simulink model "jplsetispec_thresh_rev003"  (Simulink 6.2)
settings: Solver=ode45  StartTime=0.0  StopTime=100  RelTol=1e-3
libraries: xbsIndex_r3 x776, xps_library x53, casper_library x4
(part 4 of 5)

== system jplsetispec_thresh_rev003/in/ct_pole2_snapshot/negedge ==
  In : Inport  Port=1  LatchInput=off
  Delay : xbsIndex_r3/Delay  latency=1  reg_retiming=off  explicit_period=off  period=1  en=off  accept_only_valid=off  init_zero=on  dbl_ovrd=off  show_param=off
      settings: xl_area=[0, 0, 0, 0, 0, 0, 0]
  Inverter : xbsIndex_r3/Inverter  latency=0  explicit_period=off  period=1  en=off  dbl_ovrd=off  show_param=off
      settings: xl_area=[0, 0, 0, 0, 0, 0, 0]
  Logical : xbsIndex_r3/Logical  logical_function=AND  inputs=2  precision=Full  arith_type=Unsigned  n_bits=8  bin_pt=2  align_bp=on  latency=0  explicit_period=off  period=1  en=off  dbl_ovrd=off  show_param=off
      settings: xl_area=[0, 0, 0, 0, 0, 0, 0]
  Out : Outport
  wires:
  Logical/1 -> Out/1
  In/1 -> Delay/1, Inverter/1
  Delay/1 -> Logical/1
  Inverter/1 -> Logical/2

== system jplsetispec_thresh_rev003/in/ct_pole2_snapshot/posedge ==
  In : Inport  Port=1  LatchInput=off
  Delay : xbsIndex_r3/Delay  latency=1  reg_retiming=off  explicit_period=off  period=1  en=off  accept_only_valid=off  init_zero=on  dbl_ovrd=off  show_param=off
      settings: xl_area=[0, 0, 0, 0, 0, 0, 0]
  Inverter : xbsIndex_r3/Inverter  latency=0  explicit_period=off  period=1  en=off  dbl_ovrd=off  show_param=off
      settings: xl_area=[0, 0, 0, 0, 0, 0, 0]
  Logical : xbsIndex_r3/Logical  logical_function=AND  inputs=2  precision=Full  arith_type=Unsigned  n_bits=8  bin_pt=2  align_bp=on  latency=0  explicit_period=off  period=1  en=off  dbl_ovrd=off  show_param=off
      settings: xl_area=[0, 0, 0, 0, 0, 0, 0]
  Out : Outport
  wires:
  Delay/1 -> Inverter/1
  Inverter/1 -> Logical/1
  In/1 -> Delay/1, Logical/2
  Logical/1 -> Out/1

== system jplsetispec_thresh_rev003/in/ct_pole2_snapshot/posedge1 ==
  In : Inport  Port=1  LatchInput=off
  Delay : xbsIndex_r3/Delay  latency=1  reg_retiming=off  explicit_period=off  period=1  en=off  accept_only_valid=off  init_zero=on  dbl_ovrd=off  show_param=off
      settings: xl_area=[0, 0, 0, 0, 0, 0, 0]
  Inverter : xbsIndex_r3/Inverter  latency=0  explicit_period=off  period=1  en=off  dbl_ovrd=off  show_param=off
      settings: xl_area=[0, 0, 0, 0, 0, 0, 0]
  Logical : xbsIndex_r3/Logical  logical_function=AND  inputs=2  precision=Full  arith_type=Unsigned  n_bits=8  bin_pt=2  align_bp=on  latency=0  explicit_period=off  period=1  en=off  dbl_ovrd=off  show_param=off
      settings: xl_area=[0, 0, 0, 0, 0, 0, 0]
  Out : Outport
  wires:
  Logical/1 -> Out/1
  In/1 -> Logical/2, Delay/1
  Inverter/1 -> Logical/1
  Delay/1 -> Inverter/1

== system jplsetispec_thresh_rev003/in/fft_pole1_snapshot/freeze_cntr ==
  en : Inport  Port=1  LatchInput=off
  rst : Inport  Port=2  LatchInput=off
  Constant5 : xbsIndex_r3/Constant  const=2^CounterBits - 1  equ=P=C  arith_type=Unsigned  n_bits=CounterBits  bin_pt=0  opselect=C  inp2=PCIN>>17  opr=+  inp1=P  carry=CIN  iostate=0  explicit_period=off  period=1  dbl_ovrd=off
  Counter3 : xbsIndex_r3/Counter  cnt_type=Free Running  n_bits=CounterBits  bin_pt=0  arith_type=Unsigned  start_count=0  cnt_to=1023  cnt_by_val=1  operation=Up  explicit_period=on  period=1  load_pin=off  rst=on  en=on  dbl_ovrd=off  show_param=off  use_rpm=on  gen_core=off
      settings: xl_area=[0, 0, 0, 0, 0, 0, 0]
  Inverter : xbsIndex_r3/Inverter  latency=0  explicit_period=off  period=1  en=off  dbl_ovrd=off  show_param=off
      settings: xl_area=[0, 0, 0, 0, 0, 0, 0]
  Logical1 : xbsIndex_r3/Logical  logical_function=AND  inputs=2  precision=Full  arith_type=Unsigned  n_bits=8  bin_pt=2  align_bp=on  latency=0  explicit_period=off  period=1  en=off  dbl_ovrd=off  show_param=off
      settings: xl_area=[0, 0, 0, 0, 0, 0, 0]
  Logical5 : xbsIndex_r3/Logical  logical_function=AND  inputs=2  precision=Full  arith_type=Unsigned  n_bits=8  bin_pt=2  align_bp=on  latency=0  explicit_period=off  period=1  en=off  dbl_ovrd=off  show_param=off
      settings: xl_area=[0, 0, 0, 0, 0, 0, 0]
  Relational5 : xbsIndex_r3/Relational  mode=a!=b  latency=0  explicit_period=off  period=1  en=off  dbl_ovrd=off  show_param=off
      settings: xl_area=[0, 0, 0, 0, 0, 0, 0]
  addr : Outport
  we : Outport  Port=2
  wires:
  Logical1/1 -> we/1
  Inverter/1 -> Logical1/1
  Counter3/1 -> addr/1, Relational5/1
  Constant5/1 -> Relational5/2
  Relational5/1 -> Logical5/2
  en/1 -> Logical5/1
  Logical5/1 -> Logical1/2, Counter3/2
  rst/1 -> Inverter/1, Counter3/1

== system jplsetispec_thresh_rev003/in/fft_pole1_snapshot/negedge ==
  In : Inport  Port=1  LatchInput=off
  Delay : xbsIndex_r3/Delay  latency=1  reg_retiming=off  explicit_period=off  period=1  en=off  accept_only_valid=off  init_zero=on  dbl_ovrd=off  show_param=off
      settings: xl_area=[0, 0, 0, 0, 0, 0, 0]
  Inverter : xbsIndex_r3/Inverter  latency=0  explicit_period=off  period=1  en=off  dbl_ovrd=off  show_param=off
      settings: xl_area=[0, 0, 0, 0, 0, 0, 0]
  Logical : xbsIndex_r3/Logical  logical_function=AND  inputs=2  precision=Full  arith_type=Unsigned  n_bits=8  bin_pt=2  align_bp=on  latency=0  explicit_period=off  period=1  en=off  dbl_ovrd=off  show_param=off
      settings: xl_area=[0, 0, 0, 0, 0, 0, 0]
  Out : Outport
  wires:
  Inverter/1 -> Logical/2
  Delay/1 -> Logical/1
  In/1 -> Inverter/1, Delay/1
  Logical/1 -> Out/1

== system jplsetispec_thresh_rev003/in/fft_pole1_snapshot/posedge ==
  In : Inport  Port=1  LatchInput=off
  Delay : xbsIndex_r3/Delay  latency=1  reg_retiming=off  explicit_period=off  period=1  en=off  accept_only_valid=off  init_zero=on  dbl_ovrd=off  show_param=off
      settings: xl_area=[0, 0, 0, 0, 0, 0, 0]
  Inverter : xbsIndex_r3/Inverter  latency=0  explicit_period=off  period=1  en=off  dbl_ovrd=off  show_param=off
      settings: xl_area=[0, 0, 0, 0, 0, 0, 0]
  Logical : xbsIndex_r3/Logical  logical_function=AND  inputs=2  precision=Full  arith_type=Unsigned  n_bits=8  bin_pt=2  align_bp=on  latency=0  explicit_period=off  period=1  en=off  dbl_ovrd=off  show_param=off
      settings: xl_area=[0, 0, 0, 0, 0, 0, 0]
  Out : Outport
  wires:
  Logical/1 -> Out/1
  In/1 -> Logical/2, Delay/1
  Inverter/1 -> Logical/1
  Delay/1 -> Inverter/1

== system jplsetispec_thresh_rev003/in/fft_pole1_snapshot/posedge1 ==
  In : Inport  Port=1  LatchInput=off
  Delay : xbsIndex_r3/Delay  latency=1  reg_retiming=off  explicit_period=off  period=1  en=off  accept_only_valid=off  init_zero=on  dbl_ovrd=off  show_param=off
      settings: xl_area=[0, 0, 0, 0, 0, 0, 0]
  Inverter : xbsIndex_r3/Inverter  latency=0  explicit_period=off  period=1  en=off  dbl_ovrd=off  show_param=off
      settings: xl_area=[0, 0, 0, 0, 0, 0, 0]
  Logical : xbsIndex_r3/Logical  logical_function=AND  inputs=2  precision=Full  arith_type=Unsigned  n_bits=8  bin_pt=2  align_bp=on  latency=0  explicit_period=off  period=1  en=off  dbl_ovrd=off  show_param=off
      settings: xl_area=[0, 0, 0, 0, 0, 0, 0]
  Out : Outport
  wires:
  Delay/1 -> Inverter/1
  Inverter/1 -> Logical/1
  In/1 -> Delay/1, Logical/2
  Logical/1 -> Out/1

== system jplsetispec_thresh_rev003/in/fft_pole2_snapshot/freeze_cntr ==
  en : Inport  Port=1  LatchInput=off
  rst : Inport  Port=2  LatchInput=off
  Constant5 : xbsIndex_r3/Constant  const=2^CounterBits - 1  equ=P=C  arith_type=Unsigned  n_bits=CounterBits  bin_pt=0  opselect=C  inp2=PCIN>>17  opr=+  inp1=P  carry=CIN  iostate=0  explicit_period=off  period=1  dbl_ovrd=off
  Counter3 : xbsIndex_r3/Counter  cnt_type=Free Running  n_bits=CounterBits  bin_pt=0  arith_type=Unsigned  start_count=0  cnt_to=1023  cnt_by_val=1  operation=Up  explicit_period=on  period=1  load_pin=off  rst=on  en=on  dbl_ovrd=off  show_param=off  use_rpm=on  gen_core=off
      settings: xl_area=[0, 0, 0, 0, 0, 0, 0]
  Inverter : xbsIndex_r3/Inverter  latency=0  explicit_period=off  period=1  en=off  dbl_ovrd=off  show_param=off
      settings: xl_area=[0, 0, 0, 0, 0, 0, 0]
  Logical1 : xbsIndex_r3/Logical  logical_function=AND  inputs=2  precision=Full  arith_type=Unsigned  n_bits=8  bin_pt=2  align_bp=on  latency=0  explicit_period=off  period=1  en=off  dbl_ovrd=off  show_param=off
      settings: xl_area=[0, 0, 0, 0, 0, 0, 0]
  Logical5 : xbsIndex_r3/Logical  logical_function=AND  inputs=2  precision=Full  arith_type=Unsigned  n_bits=8  bin_pt=2  align_bp=on  latency=0  explicit_period=off  period=1  en=off  dbl_ovrd=off  show_param=off
      settings: xl_area=[0, 0, 0, 0, 0, 0, 0]
  Relational5 : xbsIndex_r3/Relational  mode=a!=b  latency=0  explicit_period=off  period=1  en=off  dbl_ovrd=off  show_param=off
      settings: xl_area=[0, 0, 0, 0, 0, 0, 0]
  addr : Outport
  we : Outport  Port=2
  wires:
  rst/1 -> Counter3/1, Inverter/1
  Logical5/1 -> Counter3/2, Logical1/2
  en/1 -> Logical5/1
  Relational5/1 -> Logical5/2
  Constant5/1 -> Relational5/2
  Counter3/1 -> Relational5/1, addr/1
  Inverter/1 -> Logical1/1
  Logical1/1 -> we/1

== system jplsetispec_thresh_rev003/in/fft_pole2_snapshot/negedge ==
  In : Inport  Port=1  LatchInput=off
  Delay : xbsIndex_r3/Delay  latency=1  reg_retiming=off  explicit_period=off  period=1  en=off  accept_only_valid=off  init_zero=on  dbl_ovrd=off  show_param=off
      settings: xl_area=[0, 0, 0, 0, 0, 0, 0]
  Inverter : xbsIndex_r3/Inverter  latency=0  explicit_period=off  period=1  en=off  dbl_ovrd=off  show_param=off
      settings: xl_area=[0, 0, 0, 0, 0, 0, 0]
  Logical : xbsIndex_r3/Logical  logical_function=AND  inputs=2  precision=Full  arith_type=Unsigned  n_bits=8  bin_pt=2  align_bp=on  latency=0  explicit_period=off  period=1  en=off  dbl_ovrd=off  show_param=off
      settings: xl_area=[0, 0, 0, 0, 0, 0, 0]
  Out : Outport
  wires:
  Logical/1 -> Out/1
  In/1 -> Delay/1, Inverter/1
  Delay/1 -> Logical/1
  Inverter/1 -> Logical/2

== system jplsetispec_thresh_rev003/in/fft_pole2_snapshot/posedge ==
  In : Inport  Port=1  LatchInput=off
  Delay : xbsIndex_r3/Delay  latency=1  reg_retiming=off  explicit_period=off  period=1  en=off  accept_only_valid=off  init_zero=on  dbl_ovrd=off  show_param=off
      settings: xl_area=[0, 0, 0, 0, 0, 0, 0]
  Inverter : xbsIndex_r3/Inverter  latency=0  explicit_period=off  period=1  en=off  dbl_ovrd=off  show_param=off
      settings: xl_area=[0, 0, 0, 0, 0, 0, 0]
  Logical : xbsIndex_r3/Logical  logical_function=AND  inputs=2  precision=Full  arith_type=Unsigned  n_bits=8  bin_pt=2  align_bp=on  latency=0  explicit_period=off  period=1  en=off  dbl_ovrd=off  show_param=off
      settings: xl_area=[0, 0, 0, 0, 0, 0, 0]
  Out : Outport
  wires:
  Delay/1 -> Inverter/1
  Inverter/1 -> Logical/1
  In/1 -> Delay/1, Logical/2
  Logical/1 -> Out/1

== system jplsetispec_thresh_rev003/in/fft_pole2_snapshot/posedge1 ==
  In : Inport  Port=1  LatchInput=off
  Delay : xbsIndex_r3/Delay  latency=1  reg_retiming=off  explicit_period=off  period=1  en=off  accept_only_valid=off  init_zero=on  dbl_ovrd=off  show_param=off
      settings: xl_area=[0, 0, 0, 0, 0, 0, 0]
  Inverter : xbsIndex_r3/Inverter  latency=0  explicit_period=off  period=1  en=off  dbl_ovrd=off  show_param=off
      settings: xl_area=[0, 0, 0, 0, 0, 0, 0]
  Logical : xbsIndex_r3/Logical  logical_function=AND  inputs=2  precision=Full  arith_type=Unsigned  n_bits=8  bin_pt=2  align_bp=on  latency=0  explicit_period=off  period=1  en=off  dbl_ovrd=off  show_param=off
      settings: xl_area=[0, 0, 0, 0, 0, 0, 0]
  Out : Outport
  wires:
  Logical/1 -> Out/1
  In/1 -> Logical/2, Delay/1
  Inverter/1 -> Logical/1
  Delay/1 -> Inverter/1

== system jplsetispec_thresh_rev003/in/pulse_extender/freeze_cntr ==
  en : Inport  Port=1  LatchInput=off
  rst : Inport  Port=2  LatchInput=off
  Constant5 : xbsIndex_r3/Constant  const=2^CounterBits - 1  equ=P=C  arith_type=Unsigned  n_bits=CounterBits  bin_pt=0  opselect=C  inp2=PCIN>>17  opr=+  inp1=P  carry=CIN  iostate=0  explicit_period=off  period=1  dbl_ovrd=off
  Counter3 : xbsIndex_r3/Counter  cnt_type=Free Running  n_bits=CounterBits  bin_pt=0  arith_type=Unsigned  start_count=0  cnt_to=1023  cnt_by_val=1  operation=Up  explicit_period=on  period=1  load_pin=off  rst=on  en=on  dbl_ovrd=off  show_param=off  use_rpm=on  gen_core=off
      settings: xl_area=[0, 0, 0, 0, 0, 0, 0]
  Inverter : xbsIndex_r3/Inverter  latency=0  explicit_period=off  period=1  en=off  dbl_ovrd=off  show_param=off
      settings: xl_area=[0, 0, 0, 0, 0, 0, 0]
  Logical1 : xbsIndex_r3/Logical  logical_function=AND  inputs=2  precision=Full  arith_type=Unsigned  n_bits=8  bin_pt=2  align_bp=on  latency=0  explicit_period=off  period=1  en=off  dbl_ovrd=off  show_param=off
      settings: xl_area=[0, 0, 0, 0, 0, 0, 0]
  Logical5 : xbsIndex_r3/Logical  logical_function=AND  inputs=2  precision=Full  arith_type=Unsigned  n_bits=8  bin_pt=2  align_bp=on  latency=0  explicit_period=off  period=1  en=off  dbl_ovrd=off  show_param=off
      settings: xl_area=[0, 0, 0, 0, 0, 0, 0]
  Relational5 : xbsIndex_r3/Relational  mode=a!=b  latency=0  explicit_period=off  period=1  en=off  dbl_ovrd=off  show_param=off
      settings: xl_area=[0, 0, 0, 0, 0, 0, 0]
  addr : Outport
  we : Outport  Port=2
  wires:
  Logical1/1 -> we/1
  Inverter/1 -> Logical1/1
  Counter3/1 -> addr/1, Relational5/1
  Constant5/1 -> Relational5/2
  Relational5/1 -> Logical5/2
  en/1 -> Logical5/1
  Logical5/1 -> Logical1/2, Counter3/2
  rst/1 -> Inverter/1, Counter3/1

== system jplsetispec_thresh_rev003/in/pulse_extender/posedge ==
  In : Inport  Port=1  LatchInput=off
  Delay : xbsIndex_r3/Delay  latency=1  reg_retiming=off  explicit_period=off  period=1  en=off  accept_only_valid=off  init_zero=on  dbl_ovrd=off  show_param=off
      settings: xl_area=[0, 0, 0, 0, 0, 0, 0]
  Inverter : xbsIndex_r3/Inverter  latency=0  explicit_period=off  period=1  en=off  dbl_ovrd=off  show_param=off
      settings: xl_area=[0, 0, 0, 0, 0, 0, 0]
  Logical : xbsIndex_r3/Logical  logical_function=AND  inputs=2  precision=Full  arith_type=Unsigned  n_bits=8  bin_pt=2  align_bp=on  latency=0  explicit_period=off  period=1  en=off  dbl_ovrd=off  show_param=off
      settings: xl_area=[0, 0, 0, 0, 0, 0, 0]
  Out : Outport
  wires:
  Logical/1 -> Out/1
  In/1 -> Logical/2, Delay/1
  Inverter/1 -> Logical/1
  Delay/1 -> Inverter/1

== system jplsetispec_thresh_rev003/in/pulse_extender1/freeze_cntr ==
  en : Inport  Port=1  LatchInput=off
  rst : Inport  Port=2  LatchInput=off
  Constant5 : xbsIndex_r3/Constant  const=2^CounterBits - 1  equ=P=C  arith_type=Unsigned  n_bits=CounterBits  bin_pt=0  opselect=C  inp2=PCIN>>17  opr=+  inp1=P  carry=CIN  iostate=0  explicit_period=off  period=1  dbl_ovrd=off
  Counter3 : xbsIndex_r3/Counter  cnt_type=Free Running  n_bits=CounterBits  bin_pt=0  arith_type=Unsigned  start_count=0  cnt_to=1023  cnt_by_val=1  operation=Up  explicit_period=on  period=1  load_pin=off  rst=on  en=on  dbl_ovrd=off  show_param=off  use_rpm=on  gen_core=off
      settings: xl_area=[0, 0, 0, 0, 0, 0, 0]
  Inverter : xbsIndex_r3/Inverter  latency=0  explicit_period=off  period=1  en=off  dbl_ovrd=off  show_param=off
      settings: xl_area=[0, 0, 0, 0, 0, 0, 0]
  Logical1 : xbsIndex_r3/Logical  logical_function=AND  inputs=2  precision=Full  arith_type=Unsigned  n_bits=8  bin_pt=2  align_bp=on  latency=0  explicit_period=off  period=1  en=off  dbl_ovrd=off  show_param=off
      settings: xl_area=[0, 0, 0, 0, 0, 0, 0]
  Logical5 : xbsIndex_r3/Logical  logical_function=AND  inputs=2  precision=Full  arith_type=Unsigned  n_bits=8  bin_pt=2  align_bp=on  latency=0  explicit_period=off  period=1  en=off  dbl_ovrd=off  show_param=off
      settings: xl_area=[0, 0, 0, 0, 0, 0, 0]
  Relational5 : xbsIndex_r3/Relational  mode=a!=b  latency=0  explicit_period=off  period=1  en=off  dbl_ovrd=off  show_param=off
      settings: xl_area=[0, 0, 0, 0, 0, 0, 0]
  addr : Outport
  we : Outport  Port=2
  wires:
  Logical1/1 -> we/1
  Inverter/1 -> Logical1/1
  Counter3/1 -> addr/1, Relational5/1
  Constant5/1 -> Relational5/2
  Relational5/1 -> Logical5/2
  en/1 -> Logical5/1
  Logical5/1 -> Logical1/2, Counter3/2
  rst/1 -> Inverter/1, Counter3/1

== system jplsetispec_thresh_rev003/in/pulse_extender1/posedge ==
  In : Inport  Port=1  LatchInput=off
  Delay : xbsIndex_r3/Delay  latency=1  reg_retiming=off  explicit_period=off  period=1  en=off  accept_only_valid=off  init_zero=on  dbl_ovrd=off  show_param=off
      settings: xl_area=[0, 0, 0, 0, 0, 0, 0]
  Inverter : xbsIndex_r3/Inverter  latency=0  explicit_period=off  period=1  en=off  dbl_ovrd=off  show_param=off
      settings: xl_area=[0, 0, 0, 0, 0, 0, 0]
  Logical : xbsIndex_r3/Logical  logical_function=AND  inputs=2  precision=Full  arith_type=Unsigned  n_bits=8  bin_pt=2  align_bp=on  latency=0  explicit_period=off  period=1  en=off  dbl_ovrd=off  show_param=off
      settings: xl_area=[0, 0, 0, 0, 0, 0, 0]
  Out : Outport
  wires:
  Logical/1 -> Out/1
  In/1 -> Logical/2, Delay/1
  Inverter/1 -> Logical/1
  Delay/1 -> Inverter/1

== system jplsetispec_thresh_rev003/in/tvg/pulse_extender ==
  in : Inport  Port=1  LatchInput=off
  Constant : xbsIndex_r3/Constant  const=1  equ=P=C  arith_type=Boolean  n_bits=1  bin_pt=0  opselect=C  inp2=PCIN>>17  opr=+  inp1=P  carry=CIN  iostate=0  explicit_period=off  period=1  dbl_ovrd=off
  Constant17 : xbsIndex_r3/Constant  const=pulse_len  equ=P=C  arith_type=Unsigned  n_bits=bits  bin_pt=0  opselect=C  inp2=PCIN>>17  opr=+  inp1=P  carry=CIN  iostate=0  explicit_period=on  period=1  dbl_ovrd=off
  Logical : xbsIndex_r3/Logical  logical_function=AND  inputs=2  precision=Full  arith_type=Unsigned  n_bits=8  bin_pt=2  align_bp=on  latency=0  explicit_period=off  period=1  en=off  dbl_ovrd=off  show_param=off
      settings: xl_area=[0, 0, 0, 0, 0, 0, 0]
  Register : xbsIndex_r3/Register  init=0  reg_only_valid=off  explicit_period=off  period=1  rst=off  en=on  out_en=off  dbl_ovrd=off  show_param=off
      settings: xl_area=[0, 0, 0, 0, 0, 0, 0]
  Relational1 : xbsIndex_r3/Relational  mode=a<b  latency=0  explicit_period=off  period=1  en=off  dbl_ovrd=off  show_param=off
      settings: xl_area=[0, 0, 0, 0, 0, 0, 0]
  Terminator : Terminator
  freeze_cntr : Subsystem  mask{CounterBits=bits}
      mask prompts: CounterBits "Counter Length (2^?)"
  posedge : Subsystem  Tag=Rising Edge Detector
  out : Outport
  wires:
  Logical/1 -> out/1
  Register/1 -> Logical/2
  Relational1/1 -> Logical/1
  in/1 -> Register/2, posedge/1(In)
  Constant17/1 -> Relational1/2
  posedge/1(Out) -> freeze_cntr/2(rst)
  freeze_cntr/1(addr) -> Relational1/1
  freeze_cntr/2(we) -> Terminator/1
  Constant/1 -> Register/1, freeze_cntr/1(en)

== system jplsetispec_thresh_rev003/in/tvg1/pulse_extender ==
  in : Inport  Port=1  LatchInput=off
  Constant : xbsIndex_r3/Constant  const=1  equ=P=C  arith_type=Boolean  n_bits=1  bin_pt=0  opselect=C  inp2=PCIN>>17  opr=+  inp1=P  carry=CIN  iostate=0  explicit_period=off  period=1  dbl_ovrd=off
  Constant17 : xbsIndex_r3/Constant  const=pulse_len  equ=P=C  arith_type=Unsigned  n_bits=bits  bin_pt=0  opselect=C  inp2=PCIN>>17  opr=+  inp1=P  carry=CIN  iostate=0  explicit_period=on  period=1  dbl_ovrd=off
  Logical : xbsIndex_r3/Logical  logical_function=AND  inputs=2  precision=Full  arith_type=Unsigned  n_bits=8  bin_pt=2  align_bp=on  latency=0  explicit_period=off  period=1  en=off  dbl_ovrd=off  show_param=off
      settings: xl_area=[0, 0, 0, 0, 0, 0, 0]
  Register : xbsIndex_r3/Register  init=0  reg_only_valid=off  explicit_period=off  period=1  rst=off  en=on  out_en=off  dbl_ovrd=off  show_param=off
      settings: xl_area=[0, 0, 0, 0, 0, 0, 0]
  Relational1 : xbsIndex_r3/Relational  mode=a<b  latency=0  explicit_period=off  period=1  en=off  dbl_ovrd=off  show_param=off
      settings: xl_area=[0, 0, 0, 0, 0, 0, 0]
  Terminator : Terminator
  freeze_cntr : Subsystem  mask{CounterBits=bits}
      mask prompts: CounterBits "Counter Length (2^?)"
  posedge : Subsystem  Tag=Rising Edge Detector
  out : Outport
  wires:
  Constant/1 -> freeze_cntr/1(en), Register/1
  freeze_cntr/2(we) -> Terminator/1
  freeze_cntr/1(addr) -> Relational1/1
  posedge/1(Out) -> freeze_cntr/2(rst)
  Constant17/1 -> Relational1/2
  in/1 -> posedge/1(In), Register/2
  Relational1/1 -> Logical/1
  Register/1 -> Logical/2
  Logical/1 -> out/1

== system jplsetispec_thresh_rev003/in/tvg2/pulse_extender ==
  in : Inport  Port=1  LatchInput=off
  Constant : xbsIndex_r3/Constant  const=1  equ=P=C  arith_type=Boolean  n_bits=1  bin_pt=0  opselect=C  inp2=PCIN>>17  opr=+  inp1=P  carry=CIN  iostate=0  explicit_period=off  period=1  dbl_ovrd=off
  Constant17 : xbsIndex_r3/Constant  const=pulse_len  equ=P=C  arith_type=Unsigned  n_bits=bits  bin_pt=0  opselect=C  inp2=PCIN>>17  opr=+  inp1=P  carry=CIN  iostate=0  explicit_period=on  period=1  dbl_ovrd=off
  Logical : xbsIndex_r3/Logical  logical_function=AND  inputs=2  precision=Full  arith_type=Unsigned  n_bits=8  bin_pt=2  align_bp=on  latency=0  explicit_period=off  period=1  en=off  dbl_ovrd=off  show_param=off
      settings: xl_area=[0, 0, 0, 0, 0, 0, 0]
  Register : xbsIndex_r3/Register  init=0  reg_only_valid=off  explicit_period=off  period=1  rst=off  en=on  out_en=off  dbl_ovrd=off  show_param=off
      settings: xl_area=[0, 0, 0, 0, 0, 0, 0]
  Relational1 : xbsIndex_r3/Relational  mode=a<b  latency=0  explicit_period=off  period=1  en=off  dbl_ovrd=off  show_param=off
      settings: xl_area=[0, 0, 0, 0, 0, 0, 0]
  Terminator : Terminator
  freeze_cntr : Subsystem  mask{CounterBits=bits}
      mask prompts: CounterBits "Counter Length (2^?)"
  posedge : Subsystem  Tag=Rising Edge Detector
  out : Outport
  wires:
  Constant/1 -> freeze_cntr/1(en), Register/1
  freeze_cntr/2(we) -> Terminator/1
  freeze_cntr/1(addr) -> Relational1/1
  posedge/1(Out) -> freeze_cntr/2(rst)
  Constant17/1 -> Relational1/2
  in/1 -> posedge/1(In), Register/2
  Relational1/1 -> Logical/1
  Register/1 -> Logical/2
  Logical/1 -> out/1

== system jplsetispec_thresh_rev003/in/tvg3/pulse_extender ==
  in : Inport  Port=1  LatchInput=off
  Constant : xbsIndex_r3/Constant  const=1  equ=P=C  arith_type=Boolean  n_bits=1  bin_pt=0  opselect=C  inp2=PCIN>>17  opr=+  inp1=P  carry=CIN  iostate=0  explicit_period=off  period=1  dbl_ovrd=off
  Constant17 : xbsIndex_r3/Constant  const=pulse_len  equ=P=C  arith_type=Unsigned  n_bits=bits  bin_pt=0  opselect=C  inp2=PCIN>>17  opr=+  inp1=P  carry=CIN  iostate=0  explicit_period=on  period=1  dbl_ovrd=off
  Logical : xbsIndex_r3/Logical  logical_function=AND  inputs=2  precision=Full  arith_type=Unsigned  n_bits=8  bin_pt=2  align_bp=on  latency=0  explicit_period=off  period=1  en=off  dbl_ovrd=off  show_param=off
      settings: xl_area=[0, 0, 0, 0, 0, 0, 0]
  Register : xbsIndex_r3/Register  init=0  reg_only_valid=off  explicit_period=off  period=1  rst=off  en=on  out_en=off  dbl_ovrd=off  show_param=off
      settings: xl_area=[0, 0, 0, 0, 0, 0, 0]
  Relational1 : xbsIndex_r3/Relational  mode=a<b  latency=0  explicit_period=off  period=1  en=off  dbl_ovrd=off  show_param=off
      settings: xl_area=[0, 0, 0, 0, 0, 0, 0]
  Terminator : Terminator
  freeze_cntr : Subsystem  mask{CounterBits=bits}
      mask prompts: CounterBits "Counter Length (2^?)"
  posedge : Subsystem  Tag=Rising Edge Detector
  out : Outport
  wires:
  Logical/1 -> out/1
  Register/1 -> Logical/2
  Relational1/1 -> Logical/1
  in/1 -> Register/2, posedge/1(In)
  Constant17/1 -> Relational1/2
  posedge/1(Out) -> freeze_cntr/2(rst)
  freeze_cntr/1(addr) -> Relational1/1
  freeze_cntr/2(we) -> Terminator/1
  Constant/1 -> Register/1, freeze_cntr/1(en)

== system jplsetispec_thresh_rev003/thr/avg/Scope_Input ==
  DataA : Inport  Port=1  LatchInput=off
  DataB : Inport  Port=2  LatchInput=off
  DataC : Inport  Port=3  LatchInput=off
  Sync : Inport  Port=4  LatchInput=off
  Gateway Out{1..4} (4 alike) : xbsIndex_r3/Gateway Out  output_type=Double  nbits=8  bin_pt=6  arith_type=Boolean  quantization=Truncate  overflow=Wrap  hdl_port=off  timing_constraint=None  locs_specified=off  LOCs={}  needs_fixed_name=off  show_param=off
      settings: xl_area=[0, 0, 0, 0, 0, 0, 0]
  scope_ct_p1 : Scope  NumInputPorts=4
      settings: TimeRange=225.9933774834437  YMin=0~0~0~0  YMax=0.014~0.02~140~1
  wires:
  Sync/1 -> Gateway Out4/1
  Gateway Out4/1 -> scope_ct_p1/4
  DataC/1 -> Gateway Out3/1
  Gateway Out3/1 -> scope_ct_p1/3
  DataA/1 -> Gateway Out2/1
  Gateway Out1/1 -> scope_ct_p1/2
  DataB/1 -> Gateway Out1/1
  Gateway Out2/1 -> scope_ct_p1/1

== system jplsetispec_thresh_rev003/thr/comp1/in_fft ==
  din : Inport  Port=1  LatchInput=off
  trig : Inport  Port=2  LatchInput=off
  en : Inport  Port=3  LatchInput=off
  Constant5 : xbsIndex_r3/Constant  const=1  equ=P=C  arith_type=Boolean  n_bits=1  bin_pt=0  opselect=C  inp2=PCIN>>17  opr=+  inp1=P  carry=CIN  iostate=0  explicit_period=on  period=1  dbl_ovrd=off
  Gateway Out : xbsIndex_r3/Gateway Out  output_type=Double  nbits=8  bin_pt=6  arith_type=Boolean  quantization=Truncate  overflow=Wrap  hdl_port=off  timing_constraint=None  locs_specified=off  LOCs={}  needs_fixed_name=off  show_param=off
      settings: xl_area=[0, 0, 0, 0, 0, 0, 0]
  Gateway Out1 : xbsIndex_r3/Gateway Out  output_type=Double  nbits=8  bin_pt=6  arith_type=Boolean  quantization=Truncate  overflow=Wrap  hdl_port=off  timing_constraint=None  locs_specified=off  LOCs={}  needs_fixed_name=off  show_param=off
      settings: xl_area=[0, 0, 0, 0, 0, 0, 0]
  Logical : xbsIndex_r3/Logical  logical_function=AND  inputs=2  precision=Full  arith_type=Unsigned  n_bits=8  bin_pt=2  align_bp=on  latency=0  explicit_period=on  period=1  en=off  dbl_ovrd=off  show_param=off
      settings: xl_area=[0, 0, 0, 0, 0, 0, 0]
  Reinterpret : xbsIndex_r3/Reinterpret  force_arith_type=on  arith_type=Unsigned  force_bin_pt=on  bin_pt=0  force_valid=on
  Scope : Scope  NumInputPorts=2
      settings: YMin=-5~-5  YMax=5~5
  bram : xps_library/Shared BRAM  Tag=xps:bram  arith_type=Unsigned  addr_width=nsamples  data_width=32  data_bin_pt=0  init_vals=zeros(1,4096)  sample_rate=1
  freeze_cntr : Subsystem  mask{CounterBits=nsamples}
      mask prompts: CounterBits "Counter Length (2^?)"
  posedge : Subsystem  Tag=Rising Edge Detector
  wires:
  Gateway Out1/1 -> Scope/2
  Gateway Out/1 -> Scope/1
  bram/1 -> Gateway Out/1
  freeze_cntr/1(addr) -> bram/1
  en/1 -> Logical/1
  trig/1 -> Logical/2
  posedge/1(Out) -> freeze_cntr/2(rst)
  Logical/1 -> posedge/1(In)
  freeze_cntr/2(we) -> Gateway Out1/1, bram/3
  Constant5/1 -> freeze_cntr/1(en)
  Reinterpret/1 -> bram/2
  din/1 -> Reinterpret/1

== system jplsetispec_thresh_rev003/thr/comp1/in_thr ==
  din : Inport  Port=1  LatchInput=off
  trig : Inport  Port=2  LatchInput=off
  en : Inport  Port=3  LatchInput=off
  Constant5 : xbsIndex_r3/Constant  const=1  equ=P=C  arith_type=Boolean  n_bits=1  bin_pt=0  opselect=C  inp2=PCIN>>17  opr=+  inp1=P  carry=CIN  iostate=0  explicit_period=on  period=1  dbl_ovrd=off
  Gateway Out : xbsIndex_r3/Gateway Out  output_type=Double  nbits=8  bin_pt=6  arith_type=Boolean  quantization=Truncate  overflow=Wrap  hdl_port=off  timing_constraint=None  locs_specified=off  LOCs={}  needs_fixed_name=off  show_param=off
      settings: xl_area=[0, 0, 0, 0, 0, 0, 0]
  Gateway Out1 : xbsIndex_r3/Gateway Out  output_type=Double  nbits=8  bin_pt=6  arith_type=Boolean  quantization=Truncate  overflow=Wrap  hdl_port=off  timing_constraint=None  locs_specified=off  LOCs={}  needs_fixed_name=off  show_param=off
      settings: xl_area=[0, 0, 0, 0, 0, 0, 0]
  Logical : xbsIndex_r3/Logical  logical_function=AND  inputs=2  precision=Full  arith_type=Unsigned  n_bits=8  bin_pt=2  align_bp=on  latency=0  explicit_period=on  period=1  en=off  dbl_ovrd=off  show_param=off
      settings: xl_area=[0, 0, 0, 0, 0, 0, 0]
  Reinterpret : xbsIndex_r3/Reinterpret  force_arith_type=on  arith_type=Unsigned  force_bin_pt=on  bin_pt=0  force_valid=on
  Scope : Scope  NumInputPorts=2
      settings: YMin=-5~-5  YMax=5~5
  bram : xps_library/Shared BRAM  Tag=xps:bram  arith_type=Unsigned  addr_width=nsamples  data_width=32  data_bin_pt=0  init_vals=zeros(1,4096)  sample_rate=1
  freeze_cntr : Subsystem  mask{CounterBits=nsamples}
      mask prompts: CounterBits "Counter Length (2^?)"
  posedge : Subsystem  Tag=Rising Edge Detector
  wires:
  din/1 -> Reinterpret/1
  Reinterpret/1 -> bram/2
  Constant5/1 -> freeze_cntr/1(en)
  freeze_cntr/2(we) -> bram/3, Gateway Out1/1
  Logical/1 -> posedge/1(In)
  posedge/1(Out) -> freeze_cntr/2(rst)
  trig/1 -> Logical/2
  en/1 -> Logical/1
  freeze_cntr/1(addr) -> bram/1
  bram/1 -> Gateway Out/1
  Gateway Out/1 -> Scope/1
  Gateway Out1/1 -> Scope/2

== system jplsetispec_thresh_rev003/thr/comp1/out_event ==
  din : Inport  Port=1  LatchInput=off
  trig : Inport  Port=2  LatchInput=off
  en : Inport  Port=3  LatchInput=off
  Constant5 : xbsIndex_r3/Constant  const=1  equ=P=C  arith_type=Boolean  n_bits=1  bin_pt=0  opselect=C  inp2=PCIN>>17  opr=+  inp1=P  carry=CIN  iostate=0  explicit_period=on  period=1  dbl_ovrd=off
  Gateway Out : xbsIndex_r3/Gateway Out  output_type=Double  nbits=8  bin_pt=6  arith_type=Boolean  quantization=Truncate  overflow=Wrap  hdl_port=off  timing_constraint=None  locs_specified=off  LOCs={}  needs_fixed_name=off  show_param=off
      settings: xl_area=[0, 0, 0, 0, 0, 0, 0]
  Gateway Out1 : xbsIndex_r3/Gateway Out  output_type=Double  nbits=8  bin_pt=6  arith_type=Boolean  quantization=Truncate  overflow=Wrap  hdl_port=off  timing_constraint=None  locs_specified=off  LOCs={}  needs_fixed_name=off  show_param=off
      settings: xl_area=[0, 0, 0, 0, 0, 0, 0]
  Logical : xbsIndex_r3/Logical  logical_function=AND  inputs=2  precision=Full  arith_type=Unsigned  n_bits=8  bin_pt=2  align_bp=on  latency=0  explicit_period=on  period=1  en=off  dbl_ovrd=off  show_param=off
      settings: xl_area=[0, 0, 0, 0, 0, 0, 0]
  Reinterpret : xbsIndex_r3/Reinterpret  force_arith_type=on  arith_type=Unsigned  force_bin_pt=on  bin_pt=0  force_valid=on
  Scope : Scope  NumInputPorts=2
      settings: YMin=-5~-5  YMax=5~5
  bram : xps_library/Shared BRAM  Tag=xps:bram  arith_type=Unsigned  addr_width=nsamples  data_width=32  data_bin_pt=0  init_vals=zeros(1,4096)  sample_rate=1
  freeze_cntr : Subsystem  mask{CounterBits=nsamples}
      mask prompts: CounterBits "Counter Length (2^?)"
  posedge : Subsystem  Tag=Rising Edge Detector
  wires:
  din/1 -> Reinterpret/1
  Reinterpret/1 -> bram/2
  Constant5/1 -> freeze_cntr/1(en)
  freeze_cntr/2(we) -> bram/3, Gateway Out1/1
  Logical/1 -> posedge/1(In)
  posedge/1(Out) -> freeze_cntr/2(rst)
  trig/1 -> Logical/2
  en/1 -> Logical/1
  freeze_cntr/1(addr) -> bram/1
  bram/1 -> Gateway Out/1
  Gateway Out/1 -> Scope/1
  Gateway Out1/1 -> Scope/2

== system jplsetispec_thresh_rev003/thr/comp1/out_fft ==
  din : Inport  Port=1  LatchInput=off
  trig : Inport  Port=2  LatchInput=off
  en : Inport  Port=3  LatchInput=off
  Constant5 : xbsIndex_r3/Constant  const=1  equ=P=C  arith_type=Boolean  n_bits=1  bin_pt=0  opselect=C  inp2=PCIN>>17  opr=+  inp1=P  carry=CIN  iostate=0  explicit_period=on  period=1  dbl_ovrd=off
  Gateway Out : xbsIndex_r3/Gateway Out  output_type=Double  nbits=8  bin_pt=6  arith_type=Boolean  quantization=Truncate  overflow=Wrap  hdl_port=off  timing_constraint=None  locs_specified=off  LOCs={}  needs_fixed_name=off  show_param=off
      settings: xl_area=[0, 0, 0, 0, 0, 0, 0]
  Gateway Out1 : xbsIndex_r3/Gateway Out  output_type=Double  nbits=8  bin_pt=6  arith_type=Boolean  quantization=Truncate  overflow=Wrap  hdl_port=off  timing_constraint=None  locs_specified=off  LOCs={}  needs_fixed_name=off  show_param=off
      settings: xl_area=[0, 0, 0, 0, 0, 0, 0]
  Logical : xbsIndex_r3/Logical  logical_function=AND  inputs=2  precision=Full  arith_type=Unsigned  n_bits=8  bin_pt=2  align_bp=on  latency=0  explicit_period=on  period=1  en=off  dbl_ovrd=off  show_param=off
      settings: xl_area=[0, 0, 0, 0, 0, 0, 0]
  Reinterpret : xbsIndex_r3/Reinterpret  force_arith_type=on  arith_type=Unsigned  force_bin_pt=on  bin_pt=0  force_valid=on
  Scope : Scope  NumInputPorts=2
      settings: YMin=-5~-5  YMax=5~5
  bram : xps_library/Shared BRAM  Tag=xps:bram  arith_type=Unsigned  addr_width=nsamples  data_width=32  data_bin_pt=0  init_vals=zeros(1,4096)  sample_rate=1
  freeze_cntr : Subsystem  mask{CounterBits=nsamples}
      mask prompts: CounterBits "Counter Length (2^?)"
  posedge : Subsystem  Tag=Rising Edge Detector
  wires:
  Gateway Out1/1 -> Scope/2
  Gateway Out/1 -> Scope/1
  bram/1 -> Gateway Out/1
  freeze_cntr/1(addr) -> bram/1
  en/1 -> Logical/1
  trig/1 -> Logical/2
  posedge/1(Out) -> freeze_cntr/2(rst)
  Logical/1 -> posedge/1(In)
  freeze_cntr/2(we) -> Gateway Out1/1, bram/3
  Constant5/1 -> freeze_cntr/1(en)
  Reinterpret/1 -> bram/2
  din/1 -> Reinterpret/1

== system jplsetispec_thresh_rev003/thr/comp1/out_pfb ==
  din : Inport  Port=1  LatchInput=off
  trig : Inport  Port=2  LatchInput=off
  en : Inport  Port=3  LatchInput=off
  Constant5 : xbsIndex_r3/Constant  const=1  equ=P=C  arith_type=Boolean  n_bits=1  bin_pt=0  opselect=C  inp2=PCIN>>17  opr=+  inp1=P  carry=CIN  iostate=0  explicit_period=on  period=1  dbl_ovrd=off
  Gateway Out : xbsIndex_r3/Gateway Out  output_type=Double  nbits=8  bin_pt=6  arith_type=Boolean  quantization=Truncate  overflow=Wrap  hdl_port=off  timing_constraint=None  locs_specified=off  LOCs={}  needs_fixed_name=off  show_param=off
      settings: xl_area=[0, 0, 0, 0, 0, 0, 0]
  Gateway Out1 : xbsIndex_r3/Gateway Out  output_type=Double  nbits=8  bin_pt=6  arith_type=Boolean  quantization=Truncate  overflow=Wrap  hdl_port=off  timing_constraint=None  locs_specified=off  LOCs={}  needs_fixed_name=off  show_param=off
      settings: xl_area=[0, 0, 0, 0, 0, 0, 0]
  Logical : xbsIndex_r3/Logical  logical_function=AND  inputs=2  precision=Full  arith_type=Unsigned  n_bits=8  bin_pt=2  align_bp=on  latency=0  explicit_period=on  period=1  en=off  dbl_ovrd=off  show_param=off
      settings: xl_area=[0, 0, 0, 0, 0, 0, 0]
  Reinterpret : xbsIndex_r3/Reinterpret  force_arith_type=on  arith_type=Unsigned  force_bin_pt=on  bin_pt=0  force_valid=on
  Scope : Scope  NumInputPorts=2
      settings: YMin=-5~-5  YMax=5~5
  bram : xps_library/Shared BRAM  Tag=xps:bram  arith_type=Unsigned  addr_width=nsamples  data_width=32  data_bin_pt=0  init_vals=zeros(1,4096)  sample_rate=1
  freeze_cntr : Subsystem  mask{CounterBits=nsamples}
      mask prompts: CounterBits "Counter Length (2^?)"
  posedge : Subsystem  Tag=Rising Edge Detector
  wires:
  din/1 -> Reinterpret/1
  Reinterpret/1 -> bram/2
  Constant5/1 -> freeze_cntr/1(en)
  freeze_cntr/2(we) -> bram/3, Gateway Out1/1
  Logical/1 -> posedge/1(In)
  posedge/1(Out) -> freeze_cntr/2(rst)
  trig/1 -> Logical/2
  en/1 -> Logical/1
  freeze_cntr/1(addr) -> bram/1
  bram/1 -> Gateway Out/1
  Gateway Out/1 -> Scope/1
  Gateway Out1/1 -> Scope/2

== system jplsetispec_thresh_rev003/thr/comp1/out_pwr ==
  din : Inport  Port=1  LatchInput=off
  trig : Inport  Port=2  LatchInput=off
  en : Inport  Port=3  LatchInput=off
  Constant5 : xbsIndex_r3/Constant  const=1  equ=P=C  arith_type=Boolean  n_bits=1  bin_pt=0  opselect=C  inp2=PCIN>>17  opr=+  inp1=P  carry=CIN  iostate=0  explicit_period=on  period=1  dbl_ovrd=off
  Gateway Out : xbsIndex_r3/Gateway Out  output_type=Double  nbits=8  bin_pt=6  arith_type=Boolean  quantization=Truncate  overflow=Wrap  hdl_port=off  timing_constraint=None  locs_specified=off  LOCs={}  needs_fixed_name=off  show_param=off
      settings: xl_area=[0, 0, 0, 0, 0, 0, 0]
  Gateway Out1 : xbsIndex_r3/Gateway Out  output_type=Double  nbits=8  bin_pt=6  arith_type=Boolean  quantization=Truncate  overflow=Wrap  hdl_port=off  timing_constraint=None  locs_specified=off  LOCs={}  needs_fixed_name=off  show_param=off
      settings: xl_area=[0, 0, 0, 0, 0, 0, 0]
  Logical : xbsIndex_r3/Logical  logical_function=AND  inputs=2  precision=Full  arith_type=Unsigned  n_bits=8  bin_pt=2  align_bp=on  latency=0  explicit_period=on  period=1  en=off  dbl_ovrd=off  show_param=off
      settings: xl_area=[0, 0, 0, 0, 0, 0, 0]
  Reinterpret : xbsIndex_r3/Reinterpret  force_arith_type=on  arith_type=Unsigned  force_bin_pt=on  bin_pt=0  force_valid=on
  Scope : Scope  NumInputPorts=2
      settings: YMin=-5~-5  YMax=5~5
  bram : xps_library/Shared BRAM  Tag=xps:bram  arith_type=Unsigned  addr_width=nsamples  data_width=32  data_bin_pt=0  init_vals=zeros(1,4096)  sample_rate=1
  freeze_cntr : Subsystem  mask{CounterBits=nsamples}
      mask prompts: CounterBits "Counter Length (2^?)"
  posedge : Subsystem  Tag=Rising Edge Detector
  wires:
  Gateway Out1/1 -> Scope/2
  Gateway Out/1 -> Scope/1
  bram/1 -> Gateway Out/1
  freeze_cntr/1(addr) -> bram/1
  en/1 -> Logical/1
  trig/1 -> Logical/2
  posedge/1(Out) -> freeze_cntr/2(rst)
  Logical/1 -> posedge/1(In)
  freeze_cntr/2(we) -> Gateway Out1/1, bram/3
  Constant5/1 -> freeze_cntr/1(en)
  Reinterpret/1 -> bram/2
  din/1 -> Reinterpret/1

== system jplsetispec_thresh_rev003/thr/comp1/out_thr ==
  din : Inport  Port=1  LatchInput=off
  trig : Inport  Port=2  LatchInput=off
  en : Inport  Port=3  LatchInput=off
  Constant5 : xbsIndex_r3/Constant  const=1  equ=P=C  arith_type=Boolean  n_bits=1  bin_pt=0  opselect=C  inp2=PCIN>>17  opr=+  inp1=P  carry=CIN  iostate=0  explicit_period=on  period=1  dbl_ovrd=off
  Gateway Out : xbsIndex_r3/Gateway Out  output_type=Double  nbits=8  bin_pt=6  arith_type=Boolean  quantization=Truncate  overflow=Wrap  hdl_port=off  timing_constraint=None  locs_specified=off  LOCs={}  needs_fixed_name=off  show_param=off
      settings: xl_area=[0, 0, 0, 0, 0, 0, 0]
  Gateway Out1 : xbsIndex_r3/Gateway Out  output_type=Double  nbits=8  bin_pt=6  arith_type=Boolean  quantization=Truncate  overflow=Wrap  hdl_port=off  timing_constraint=None  locs_specified=off  LOCs={}  needs_fixed_name=off  show_param=off
      settings: xl_area=[0, 0, 0, 0, 0, 0, 0]
  Logical : xbsIndex_r3/Logical  logical_function=AND  inputs=2  precision=Full  arith_type=Unsigned  n_bits=8  bin_pt=2  align_bp=on  latency=0  explicit_period=on  period=1  en=off  dbl_ovrd=off  show_param=off
      settings: xl_area=[0, 0, 0, 0, 0, 0, 0]
  Reinterpret : xbsIndex_r3/Reinterpret  force_arith_type=on  arith_type=Unsigned  force_bin_pt=on  bin_pt=0  force_valid=on
  Scope : Scope  NumInputPorts=2
      settings: YMin=-5~-5  YMax=5~5
  bram : xps_library/Shared BRAM  Tag=xps:bram  arith_type=Unsigned  addr_width=nsamples  data_width=32  data_bin_pt=0  init_vals=zeros(1,4096)  sample_rate=1
  freeze_cntr : Subsystem  mask{CounterBits=nsamples}
      mask prompts: CounterBits "Counter Length (2^?)"
  posedge : Subsystem  Tag=Rising Edge Detector
  wires:
  din/1 -> Reinterpret/1
  Reinterpret/1 -> bram/2
  Constant5/1 -> freeze_cntr/1(en)
  freeze_cntr/2(we) -> bram/3, Gateway Out1/1
  Logical/1 -> posedge/1(In)
  posedge/1(Out) -> freeze_cntr/2(rst)
  trig/1 -> Logical/2
  en/1 -> Logical/1
  freeze_cntr/1(addr) -> bram/1
  bram/1 -> Gateway Out/1
  Gateway Out/1 -> Scope/1
  Gateway Out1/1 -> Scope/2

== system jplsetispec_thresh_rev003/thr/comp2/Scope_Input ==
  DataA : Inport  Port=1  LatchInput=off
  DataB : Inport  Port=2  LatchInput=off
  DataC : Inport  Port=3  LatchInput=off
  Sync : Inport  Port=4  LatchInput=off
  Gateway Out{1..4} (4 alike) : xbsIndex_r3/Gateway Out  output_type=Double  nbits=8  bin_pt=6  arith_type=Boolean  quantization=Truncate  overflow=Wrap  hdl_port=off  timing_constraint=None  locs_specified=off  LOCs={}  needs_fixed_name=off  show_param=off
      settings: xl_area=[0, 0, 0, 0, 0, 0, 0]
  scope_ct_p1 : Scope  NumInputPorts=4
      settings: TimeRange=225.9933774834437  YMin=0~0~0~0  YMax=0.014~0.02~140~1
  wires:
  Gateway Out2/1 -> scope_ct_p1/1
  DataB/1 -> Gateway Out1/1
  Gateway Out1/1 -> scope_ct_p1/2
  DataA/1 -> Gateway Out2/1
  Gateway Out3/1 -> scope_ct_p1/3
  DataC/1 -> Gateway Out3/1
  Gateway Out4/1 -> scope_ct_p1/4
  Sync/1 -> Gateway Out4/1

== system jplsetispec_thresh_rev003/thr/comp2/Scope_Output ==
  DataA : Inport  Port=1  LatchInput=off
  DataB : Inport  Port=2  LatchInput=off
  DataC : Inport  Port=3  LatchInput=off
  DataD : Inport  Port=4  LatchInput=off
  DataE : Inport  Port=5  LatchInput=off
  "DataF " : Inport  Port=6  LatchInput=off
  "DataG " : Inport  Port=7  LatchInput=off
  Gateway Out{1..7} (7 alike) : xbsIndex_r3/Gateway Out  output_type=Double  nbits=8  bin_pt=6  arith_type=Boolean  quantization=Truncate  overflow=Wrap  hdl_port=off  timing_constraint=None  locs_specified=off  LOCs={}  needs_fixed_name=off  show_param=off
      settings: xl_area=[0, 0, 0, 0, 0, 0, 0]
  Scope_output : Scope  NumInputPorts=7
      settings: TimeRange=152.1280625333588  YMin=0~0~0~0~0~0~0  YMax=1~0.01~40~150~0.01~1~1
  wires:
  DataD/1 -> Gateway Out4/1
  DataC/1 -> Gateway Out3/1
  DataA/1 -> Gateway Out2/1
  DataB/1 -> Gateway Out1/1
  DataE/1 -> Gateway Out5/1
  "DataF "/1 -> Gateway Out6/1
  "DataG "/1 -> Gateway Out7/1
  Gateway Out4/1 -> Scope_output/4
  Gateway Out3/1 -> Scope_output/3
  Gateway Out1/1 -> Scope_output/2
  Gateway Out2/1 -> Scope_output/1
  Gateway Out5/1 -> Scope_output/5
  Gateway Out6/1 -> Scope_output/6
  Gateway Out7/1 -> Scope_output/7

== system jplsetispec_thresh_rev003/thr/ct_power/Scope_Input ==
  DataA : Inport  Port=1  LatchInput=off
  DataB : Inport  Port=2  LatchInput=off
  DataC : Inport  Port=3  LatchInput=off
  Sync : Inport  Port=4  LatchInput=off
  Gateway Out{1..4} (4 alike) : xbsIndex_r3/Gateway Out  output_type=Double  nbits=8  bin_pt=6  arith_type=Boolean  quantization=Truncate  overflow=Wrap  hdl_port=off  timing_constraint=None  locs_specified=off  LOCs={}  needs_fixed_name=off  show_param=off
      settings: xl_area=[0, 0, 0, 0, 0, 0, 0]
  scope_ct_p1 : Scope  NumInputPorts=4
      settings: TimeRange=225.9933774834437  YMin=0~0~0~0  YMax=0.014~0.02~140~1
  wires:
  Sync/1 -> Gateway Out4/1
  Gateway Out4/1 -> scope_ct_p1/4
  DataC/1 -> Gateway Out3/1
  Gateway Out3/1 -> scope_ct_p1/3
  DataA/1 -> Gateway Out2/1
  Gateway Out1/1 -> scope_ct_p1/2
  DataB/1 -> Gateway Out1/1
  Gateway Out2/1 -> scope_ct_p1/1

== system jplsetispec_thresh_rev003/thr/fft_power/Scope_Input ==
  DataA : Inport  Port=1  LatchInput=off
  DataB : Inport  Port=2  LatchInput=off
  DataC : Inport  Port=3  LatchInput=off
  Sync : Inport  Port=4  LatchInput=off
  Gateway Out{1..4} (4 alike) : xbsIndex_r3/Gateway Out  output_type=Double  nbits=8  bin_pt=6  arith_type=Boolean  quantization=Truncate  overflow=Wrap  hdl_port=off  timing_constraint=None  locs_specified=off  LOCs={}  needs_fixed_name=off  show_param=off
      settings: xl_area=[0, 0, 0, 0, 0, 0, 0]
  scope_ct_p1 : Scope  NumInputPorts=4
      settings: TimeRange=225.9933774834437  YMin=0~0~0~0  YMax=0.014~0.02~140~1
  wires:
  Sync/1 -> Gateway Out4/1
  Gateway Out4/1 -> scope_ct_p1/4
  DataC/1 -> Gateway Out3/1
  Gateway Out3/1 -> scope_ct_p1/3
  DataA/1 -> Gateway Out2/1
  Gateway Out1/1 -> scope_ct_p1/2
  DataB/1 -> Gateway Out1/1
  Gateway Out2/1 -> scope_ct_p1/1

== system jplsetispec_thresh_rev003/thr/scale/Scope_Input ==
  DataA : Inport  Port=1  LatchInput=off
  DataB : Inport  Port=2  LatchInput=off
  DataC : Inport  Port=3  LatchInput=off
  Sync : Inport  Port=4  LatchInput=off
  Gateway Out{1..4} (4 alike) : xbsIndex_r3/Gateway Out  output_type=Double  nbits=8  bin_pt=6  arith_type=Boolean  quantization=Truncate  overflow=Wrap  hdl_port=off  timing_constraint=None  locs_specified=off  LOCs={}  needs_fixed_name=off  show_param=off
      settings: xl_area=[0, 0, 0, 0, 0, 0, 0]
  scope_ct_p1 : Scope  NumInputPorts=4
      settings: TimeRange=225.9933774834437  YMin=0~0~0~0  YMax=0.014~0.02~140~1
  wires:
  Sync/1 -> Gateway Out4/1
  Gateway Out4/1 -> scope_ct_p1/4
  DataC/1 -> Gateway Out3/1
  Gateway Out3/1 -> scope_ct_p1/3
  DataA/1 -> Gateway Out2/1
  Gateway Out1/1 -> scope_ct_p1/2
  DataB/1 -> Gateway Out1/1
  Gateway Out2/1 -> scope_ct_p1/1

== system jplsetispec_thresh_rev003/thr/scale1_snap/freeze_cntr ==
  en : Inport  Port=1  LatchInput=off
  rst : Inport  Port=2  LatchInput=off
  Constant5 : xbsIndex_r3/Constant  const=2^CounterBits - 1  equ=P=C  arith_type=Unsigned  n_bits=CounterBits  bin_pt=0  opselect=C  inp2=PCIN>>17  opr=+  inp1=P  carry=CIN  iostate=0  explicit_period=off  period=1  dbl_ovrd=off
  Counter3 : xbsIndex_r3/Counter  cnt_type=Free Running  n_bits=CounterBits  bin_pt=0  arith_type=Unsigned  start_count=0  cnt_to=1023  cnt_by_val=1  operation=Up  explicit_period=on  period=1  load_pin=off  rst=on  en=on  dbl_ovrd=off  show_param=off  use_rpm=on  gen_core=off
      settings: xl_area=[0, 0, 0, 0, 0, 0, 0]
  Inverter : xbsIndex_r3/Inverter  latency=0  explicit_period=off  period=1  en=off  dbl_ovrd=off  show_param=off
      settings: xl_area=[0, 0, 0, 0, 0, 0, 0]
  Logical1 : xbsIndex_r3/Logical  logical_function=AND  inputs=2  precision=Full  arith_type=Unsigned  n_bits=8  bin_pt=2  align_bp=on  latency=0  explicit_period=off  period=1  en=off  dbl_ovrd=off  show_param=off
      settings: xl_area=[0, 0, 0, 0, 0, 0, 0]
  Logical5 : xbsIndex_r3/Logical  logical_function=AND  inputs=2  precision=Full  arith_type=Unsigned  n_bits=8  bin_pt=2  align_bp=on  latency=0  explicit_period=off  period=1  en=off  dbl_ovrd=off  show_param=off
      settings: xl_area=[0, 0, 0, 0, 0, 0, 0]
  Relational5 : xbsIndex_r3/Relational  mode=a!=b  latency=0  explicit_period=off  period=1  en=off  dbl_ovrd=off  show_param=off
      settings: xl_area=[0, 0, 0, 0, 0, 0, 0]
  addr : Outport
  we : Outport  Port=2
  wires:
  Logical1/1 -> we/1
  Inverter/1 -> Logical1/1
  Counter3/1 -> addr/1, Relational5/1
  Constant5/1 -> Relational5/2
  Relational5/1 -> Logical5/2
  en/1 -> Logical5/1
  Logical5/1 -> Logical1/2, Counter3/2
  rst/1 -> Inverter/1, Counter3/1

== system jplsetispec_thresh_rev003/thr/scale1_snap/negedge ==
  In : Inport  Port=1  LatchInput=off
  Delay : xbsIndex_r3/Delay  latency=1  reg_retiming=off  explicit_period=off  period=1  en=off  accept_only_valid=off  init_zero=on  dbl_ovrd=off  show_param=off
      settings: xl_area=[0, 0, 0, 0, 0, 0, 0]
  Inverter : xbsIndex_r3/Inverter  latency=0  explicit_period=off  period=1  en=off  dbl_ovrd=off  show_param=off
      settings: xl_area=[0, 0, 0, 0, 0, 0, 0]
  Logical : xbsIndex_r3/Logical  logical_function=AND  inputs=2  precision=Full  arith_type=Unsigned  n_bits=8  bin_pt=2  align_bp=on  latency=0  explicit_period=off  period=1  en=off  dbl_ovrd=off  show_param=off
      settings: xl_area=[0, 0, 0, 0, 0, 0, 0]
  Out : Outport
  wires:
  Inverter/1 -> Logical/2
  Delay/1 -> Logical/1
  In/1 -> Inverter/1, Delay/1
  Logical/1 -> Out/1

== system jplsetispec_thresh_rev003/thr/scale1_snap/posedge ==
  In : Inport  Port=1  LatchInput=off
  Delay : xbsIndex_r3/Delay  latency=1  reg_retiming=off  explicit_period=off  period=1  en=off  accept_only_valid=off  init_zero=on  dbl_ovrd=off  show_param=off
      settings: xl_area=[0, 0, 0, 0, 0, 0, 0]
  Inverter : xbsIndex_r3/Inverter  latency=0  explicit_period=off  period=1  en=off  dbl_ovrd=off  show_param=off
      settings: xl_area=[0, 0, 0, 0, 0, 0, 0]
  Logical : xbsIndex_r3/Logical  logical_function=AND  inputs=2  precision=Full  arith_type=Unsigned  n_bits=8  bin_pt=2  align_bp=on  latency=0  explicit_period=off  period=1  en=off  dbl_ovrd=off  show_param=off
      settings: xl_area=[0, 0, 0, 0, 0, 0, 0]
  Out : Outport
  wires:
  Logical/1 -> Out/1
  In/1 -> Logical/2, Delay/1
  Inverter/1 -> Logical/1
  Delay/1 -> Inverter/1

== system jplsetispec_thresh_rev003/thr/scale1_snap/posedge1 ==
  In : Inport  Port=1  LatchInput=off
  Delay : xbsIndex_r3/Delay  latency=1  reg_retiming=off  explicit_period=off  period=1  en=off  accept_only_valid=off  init_zero=on  dbl_ovrd=off  show_param=off
      settings: xl_area=[0, 0, 0, 0, 0, 0, 0]
  Inverter : xbsIndex_r3/Inverter  latency=0  explicit_period=off  period=1  en=off  dbl_ovrd=off  show_param=off
      settings: xl_area=[0, 0, 0, 0, 0, 0, 0]
  Logical : xbsIndex_r3/Logical  logical_function=AND  inputs=2  precision=Full  arith_type=Unsigned  n_bits=8  bin_pt=2  align_bp=on  latency=0  explicit_period=off  period=1  en=off  dbl_ovrd=off  show_param=off
      settings: xl_area=[0, 0, 0, 0, 0, 0, 0]
  Out : Outport
  wires:
  Delay/1 -> Inverter/1
  Inverter/1 -> Logical/1
  In/1 -> Delay/1, Logical/2
  Logical/1 -> Out/1
